simulink model "PI_controller"  (R2024a)
settings: Solver=FixedStepAuto  StartTime=0.0  StopTime=20.0  FixedStep=0.01  RelTol=1e-3
settings Model: Creator=VKIST  LastModifiedBy=TRUONG GIANG
settings DebuggingCC: UnconnectedInputMsg=warning  UnconnectedOutputMsg=warning  UnconnectedLineMsg=warning
settings ModelReferenceCC: EnableRefExpFcnMdlSchedulingChecks=on
settings RTWCC: GPUComputeCapability=3.5  DLArmComputeVersion=19.05

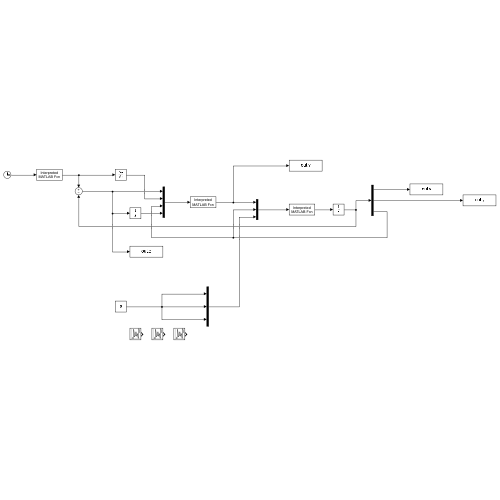
[thumbnail: Simulink's stored preview of the top-level diagram]
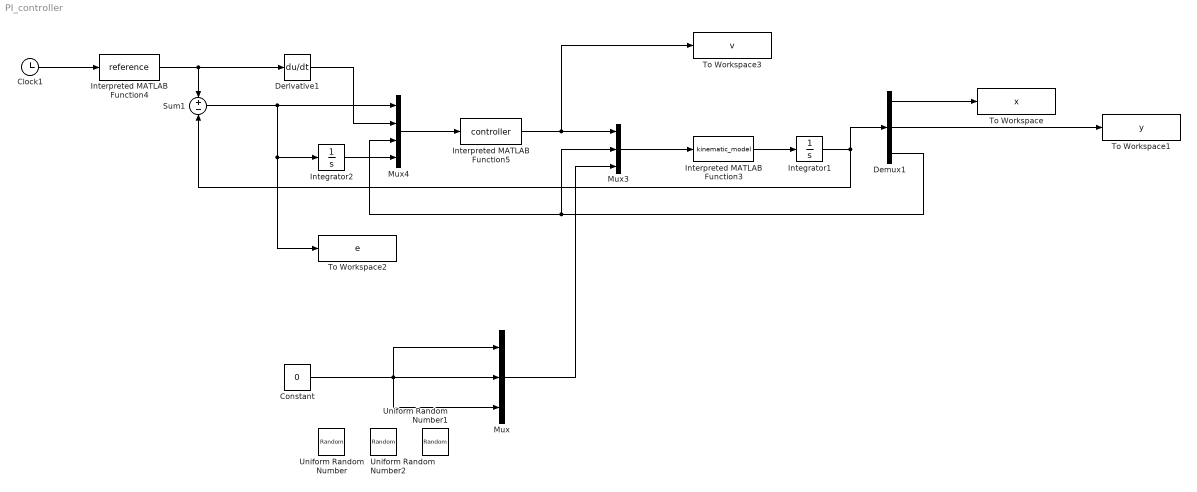
== system PI_controller ==
  Clock1 : Clock
  Constant : Constant  Value=0
  Demux1 : Demux  Outputs=3
  Derivative1 : Derivative
  Integrator1 : Integrator
  Integrator2 : Integrator
  Interpreted MATLAB Function3 : MATLABFcn  MATLABFcn=kinematic_model  OutputDimensions=3
  Interpreted MATLAB Function4 : MATLABFcn  MATLABFcn=reference  OutputDimensions=3
  Interpreted MATLAB Function5 : MATLABFcn  MATLABFcn=controller  OutputDimensions=3
  Mux : Mux  Inputs=3
  Mux3 : Mux  Inputs=3
  Mux4 : Mux
  Sum1 : Sum  Inputs=+-
  To Workspace : ToWorkspace  VariableName=x  SampleTime=-1
      settings: Save2DSignal=2-D array (concatenate along first dimension)
  To Workspace1 : ToWorkspace  VariableName=y  SampleTime=-1
      settings: Save2DSignal=2-D array (concatenate along first dimension)
  To Workspace2 : ToWorkspace  VariableName=e  SaveFormat=Timeseries  SampleTime=-1
      settings: Save2DSignal=2-D array (concatenate along first dimension)
  To Workspace3 : ToWorkspace  VariableName=v  SaveFormat=Timeseries  SampleTime=-1
      settings: Save2DSignal=2-D array (concatenate along first dimension)
  Uniform Random Number : UniformRandomNumber  SampleTime=0.1
  Uniform Random Number1 : UniformRandomNumber  SampleTime=0.1
  Uniform Random Number2 : UniformRandomNumber  SampleTime=0.1
  wires:
  Demux1/3 -> Mux3/2, Mux4/3
  Interpreted MATLAB Function5/1 -> Mux3/1, To Workspace3/1
  Demux1/1 -> To Workspace/1
  Integrator1/1 -> Sum1/2, Demux1/1
  Interpreted MATLAB Function4/1 -> Sum1/1, Derivative1/1
  Clock1/1 -> Interpreted MATLAB Function4/1
  Interpreted MATLAB Function3/1 -> Integrator1/1
  Mux4/1 -> Interpreted MATLAB Function5/1
  Sum1/1 -> To Workspace2/1, Integrator2/1, Mux4/1
  Mux3/1 -> Interpreted MATLAB Function3/1
  Derivative1/1 -> Mux4/2
  Demux1/2 -> To Workspace1/1
  Integrator2/1 -> Mux4/4
  Mux/1 -> Mux3/3
  Constant/1 -> Mux/1, Mux/2, Mux/3
